simulink model "piston_cylinder_deneme_mixxxx"  (R2022b)
settings: Solver=VariableStepAuto  StartTime=0.0  StopTime=7  RelTol=1e-3
undefined symbols (not defined in the file): X, Y, Z
libraries: sm_lib x45, nesl_utility x24, simulink x8, sh_lib x5, fl_lib x5
(part 4 of 4)

== matlab function piston_cylinder_deneme_mixxxx/MATLAB Function ==
  data: time input; y output; twist2 input
function y = fcn(time,twist2)
mode = rem(time,0.987);
if mode < 0.987/2
    y = twist2;
else
    y = 0;
end
end

== matlab function piston_cylinder_deneme_mixxxx/MATLAB Function4 ==
  data: time input; y output; twist input
function y = fcn(time,twist)
mode = rem(time,0.987);
if mode < 0.987/2
    y = twist;
else
    y = 0;
end
end

== matlab function piston_cylinder_deneme_mixxxx/Healthy Left Leg/MATLAB Function ==
  data: time input; y output
function y = ankle_theta(time)
	y = +0.120*cos(-7*2*pi*time+3.065)+0.334*cos(-6*2*pi*time+1.942)+0.479*cos(-5*2*pi*time+-2.193)+1.331*cos(-4*2*pi*time+2.911)+1.098*cos(-3*2*pi*time+-2.580)+3.787*cos(-2*2*pi*time+-3.020)+2.428*cos(-1*2*pi*time+-2.383)+1.399*cos(0*2*pi*time+3.142)+2.428*cos(1*2*pi*time+2.383)+3.787*cos(2*2*pi*time+3.020)+1.098*cos(3*2*pi*time+2.580)+1.331*cos(4*2*pi*time+-2.911)+0.479*cos(5*2*pi*time+2.193)+0.334*cos(6*2*pi*time+-1.942)+0.120*cos(7*2*pi*time+-3.065);
end

== matlab function piston_cylinder_deneme_mixxxx/Prosthesis Leg/MATLAB Function2 ==
  data: x input; y output
function y = fcn(x)
a0 =      0.8196  
a1 =      -0.769  
b1 =      -1.085  
a2 =     -0.1778  
b2 =      0.6378  
a3 =     0.08544  
b3 =     -0.1232  
a4 =    0.003099  
b4 =      0.1184  
a5 =     0.03895  
b5 =    -0.04715  
a6 =   -0.002965  
b6 =    0.009594  
a7 =    0.009704  
b7 =   -0.006175  
a8 =  -0.0006199  
b8 =   -0.007626  
w =     0.07303  
y = a0 + a1*cos(x*w) + b1*sin(x*w) + a2*cos(2*x*w) + b2*sin(2*x*w) + a3*cos(3*x*w) + b3*sin(3*x*w) + a4*cos(4*x*w) + b4*sin(4*x*w) + a5*cos(5*x*w) + b5*sin(5*x*w) + a6*cos(6*x*w) + b6*sin(6*x*w) + a7*cos(7*x*w) + b7*sin(7*x*w) + a8*cos(8*x*w) + b8*sin(8*x*w)

== matlab function piston_cylinder_deneme_mixxxx/Healthy Left Leg/MATLAB Function4 ==
  data: knee_angle output; time input
function knee_angle = fcn( time)

time = (time+(0.987/2))
knee_angle = +0.104*cos(-7*2*pi*time+-2.019)+0.156*cos(-6*2*pi*time+2.272)+0.246*cos(-5*2*pi*time+2.119)+0.557*cos(-4*2*pi*time+-0.156)+2.099*cos(-3*2*pi*time+2.573)+9.262*cos(-2*2*pi*time+1.156)+11.856*cos(-1*2*pi*time+0.545)+22.700*cos(0*2*pi*time+0.000)+11.856*cos(1*2*pi*time+-0.545)+9.262*cos(2*2*pi*time+-1.156)+2.099*cos(3*2*pi*time+-2.573)+0.557*cos(4*2*pi*time+0.156)+0.246*cos(5*2*pi*time+-2.119)+0.156*cos(6*2*pi*time+-2.272)+0.104*cos(7*2*pi*time+2.019)
